simulink model "AE4"  (R2015a)
settings: Solver=ode45  StartTime=0.0  StopTime=0.1  RelTol=1e-3
libraries: dspsrcs4 x3, dsparch4 x2, dspsnks4 x1
settings Model: Creator=aluno  LastModifiedBy=aluno

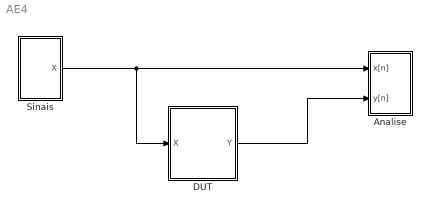
== system AE4 ==
  Analise : Subsystem
  DUT : Subsystem
  Sinais : Subsystem  mask{fa=8000, spf=256, fonte=1, v1=0.5, f1=2500}
      mask prompts: fa "Freq. amostragem (Hz)"; spf "Amostras por frame"; fonte "Fonte (switch)"; v1 "Amplitude da senoide"; f1 "Freq. da senoide"
      mask TypeOptions fonte: 1 | 2 | 3 | 4 | 5
  wires:
  Sinais/1(X) -> DUT/1(X), Analise/1(x[n])
  DUT/1(Y) -> Analise/2(y[n])

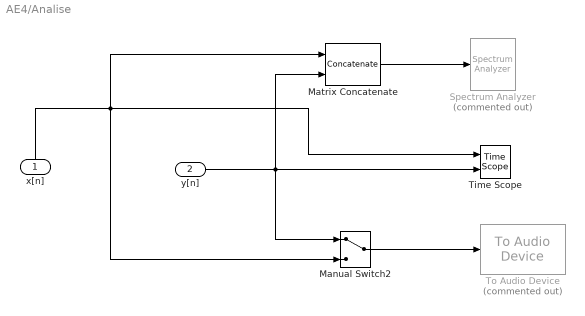
== system AE4/Analise ==
  x[n] : Inport
  y[n] : Inport  Port=2
  Manual Switch2 : ManualSwitch
  Matrix Concatenate : Concatenate  Mode=Multidimensional array  ConcatenateDimension=2
  Spectrum Analyzer : SpectrumAnalyzer  Commented=on
  Time Scope : TimeScope  DefaultConfigurationName=spbscopes.TimeScopeBlockCfg  NumInputPorts=2
  To Audio Device : dspsnks4/To Audio Device  Commented=on  deviceName=Default  inheritSampleRate=on  sampleRate=44100  deviceDatatype=Determine from input data type  autoBufferSize=on  bufferSize=4096  queueDuration=1.0  defaultOutputChannelMapping=on  outputChannelMapping=1:2  outputNumUnderrunSamples=off
  wires:
  Matrix Concatenate/1 -> Spectrum Analyzer/1
  x[n]/1 -> Manual Switch2/2, Time Scope/1, Matrix Concatenate/1
  y[n]/1 -> Manual Switch2/1, Matrix Concatenate/2, Time Scope/2
  Manual Switch2/1 -> To Audio Device/1

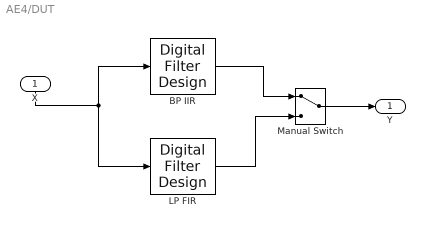
== system AE4/DUT ==
  X : Inport
  BP IIR : dsparch4/Digital Filter Design  mwdsp_browser_bugfix_var=off
  LP FIR : dsparch4/Digital Filter Design  mwdsp_browser_bugfix_var=off
  Manual Switch : ManualSwitch
  Y : Outport
  wires:
  BP IIR/1 -> Manual Switch/1
  LP FIR/1 -> Manual Switch/2
  Manual Switch/1 -> Y/1
  X/1 -> LP FIR/1, BP IIR/1

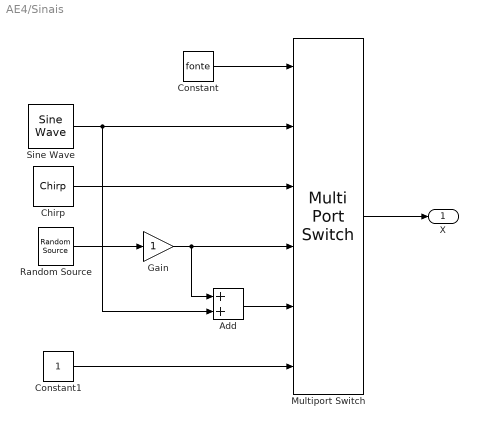
== system AE4/Sinais ==
  Add : Sum
  Chirp : dspsrcs4/Chirp  sweep=Linear  mode=Unidirectional  f0=1  f1=fa/2  t1=2  Tsweep=2  phase=0  Ts=1/fa  spf=spf  datatype=Double
  Constant : Constant  Value=fonte
  Constant1 : Constant
  Gain : Gain
  Multiport Switch : MultiPortSwitch  Inputs=5
  Random Source : dspsrcs4/Random Source  SrcType=Uniform  NormMethod=Ziggurat  CltLength=12  MinVal=-1  MaxVal=1  MeanVal=0  VarVal=1  RepMode=Not repeatable  rawSeed=1  IsInherit=off  SampMode=Discrete  SampTime=1/fa  SampFrame=spf  DataType=Double  OutComplex=Real
  Sine Wave : dspsrcs4/Sine Wave  Amplitude=v1  Frequency=f1  Phase=0  SampleMode=Discrete  OutComplex=Real  CompMethod=Trigonometric fcn  TableSize=Speed  SampleTime=1/fa  SamplesPerFrame=spf  ResetState=Restart at time zero  dataType=double  wordLen=16  udDataType=sfix(16)  fracBitsMode=Best precision  numFracBits=15  OutDataTypeStr=double  LastOutDataTypeStr=double
  X : Outport
  wires:
  Gain/1 -> Add/1, Multiport Switch/4
  Chirp/1 -> Multiport Switch/3
  Sine Wave/1 -> Add/2, Multiport Switch/2
  Multiport Switch/1 -> X/1
  Constant/1 -> Multiport Switch/1
  Add/1 -> Multiport Switch/5
  Constant1/1 -> Multiport Switch/6
  Random Source/1 -> Gain/1
